simulink model "dbsim"  (R2024b)
settings: Solver=VariableStepAuto  StartTime=tspan(1)  StopTime=tspan(2)  RelTol=1e-3
values from neighbouring files (symbols this model uses):
  DbDTFReg = DBRegRest(dtf, u_lim)    [main.m]
  RegARMAX = DBRegRest(tfarmax, u_lim)    [main.m]
  RegARX = DBRegRest(tfarx, u_lim)    [main.m]
  usim = 1    [main.m]
  ut = [1 5]    [main.m]
undefined symbols (not defined in the file or in its folder): dtf, tfarmax, tfarx
settings Model: Creator=markminerov  LastModifiedBy=markminerov
settings DebuggingCC: AlgebraicLoopMsg=none

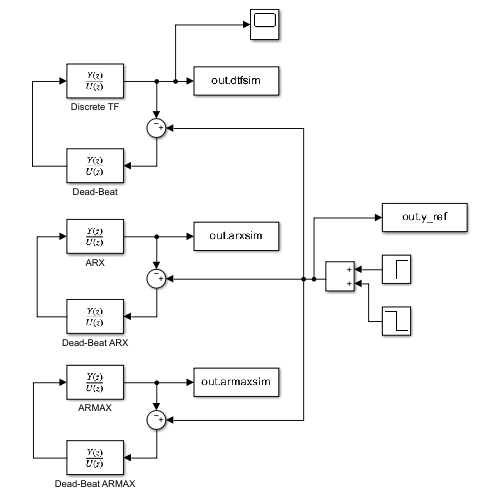
[thumbnail: Simulink's stored preview of the top-level diagram]
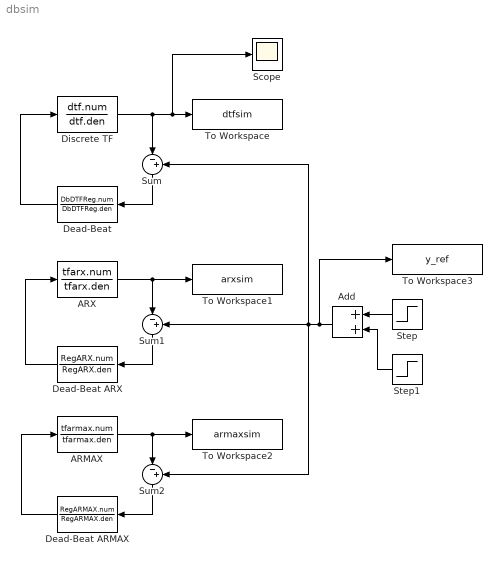
== system dbsim ==
  ARMAX : DiscreteTransferFcn  Numerator=tfarmax.num  Denominator=tfarmax.den
  ARX : DiscreteTransferFcn  Numerator=tfarx.num  Denominator=tfarx.den
  Add : Sum
  Dead-Beat : DiscreteTransferFcn  Numerator=DbDTFReg.num  Denominator=DbDTFReg.den
  Dead-Beat ARMAX : DiscreteTransferFcn  Numerator=RegARMAX.num  Denominator=RegARMAX.den
  Dead-Beat ARX : DiscreteTransferFcn  Numerator=RegARX.num  Denominator=RegARX.den
  Discrete TF : DiscreteTransferFcn  Numerator=dtf.num  Denominator=dtf.den
  Scope : Scope
  Step : Step  Time=ut(1)  After=usim  SampleTime=0
  Step1 : Step  Time=ut(2)  After=-usim  SampleTime=0
  Sum : Sum  Inputs=|-+
  Sum1 : Sum  Inputs=|-+
  Sum2 : Sum  Inputs=|-+
  To Workspace : ToWorkspace  VariableName=dtfsim  SaveFormat=Timeseries  SampleTime=-1
  To Workspace1 : ToWorkspace  VariableName=arxsim  SaveFormat=Timeseries  SampleTime=-1
  To Workspace2 : ToWorkspace  VariableName=armaxsim  SaveFormat=Timeseries  SampleTime=-1
  To Workspace3 : ToWorkspace  VariableName=y_ref  SaveFormat=Timeseries  SampleTime=-1
  wires:
  Sum1/1 -> Dead-Beat ARX/1
  Dead-Beat ARX/1 -> ARX/1
  ARX/1 -> Sum1/1, To Workspace1/1
  Sum2/1 -> Dead-Beat ARMAX/1
  Dead-Beat ARMAX/1 -> ARMAX/1
  ARMAX/1 -> To Workspace2/1, Sum2/1
  Sum/1 -> Dead-Beat/1
  Dead-Beat/1 -> Discrete TF/1
  Discrete TF/1 -> Scope/1, To Workspace/1, Sum/1
  Add/1 -> To Workspace3/1, Sum2/2, Sum1/2, Sum/2
  Step/1 -> Add/1
  Step1/1 -> Add/2
